simulink library "INT_IAirHt_VD"  (R2016b)
settings: Solver=VariableStepAuto  StartTime=0.0  StopTime=10.0  RelTol=1e-3
settings Model: Creator=Wei Liang  LastModifiedBy=Wei Liang

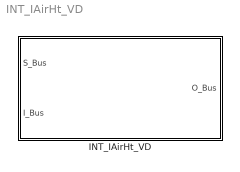
== system INT_IAirHt_VD ==
  INT_IAirHt_VD : Subsystem

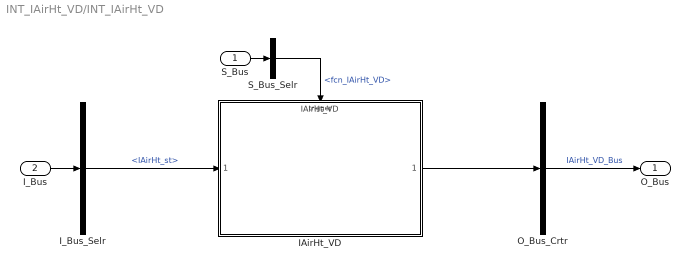
== system INT_IAirHt_VD/INT_IAirHt_VD ==
  S_Bus : Inport
  I_Bus : Inport  Port=2
  IAirHt_VD : ModelReference  ModelNameDialog=IAirHt_VD  SimulationMode=Normal  ModelReferenceVersion=1.2  TriggerPortName=function  TriggerPortTriggerType=function-call  TriggerPortStatesWhenEnabling=held
  I_Bus_Selr : BusSelector  OutputSignals=IAirHt_st
  O_Bus_Crtr : BusCreator  Inputs=1
  S_Bus_Selr : BusSelector  OutputSignals=fcn_IAirHt_VD
  O_Bus : Outport
  wires:
  S_Bus_Selr/1 -> IAirHt_VD/Trigger  "<fcn_IAirHt_VD>"
  S_Bus/1 -> S_Bus_Selr/1
  I_Bus/1 -> I_Bus_Selr/1
  I_Bus_Selr/1 -> IAirHt_VD/1  "<IAirHt_st>"
  O_Bus_Crtr/1 -> O_Bus/1  "IAirHt_VD_Bus"
  IAirHt_VD/1 -> O_Bus_Crtr/1
